simulink library "starslibAirData"  (R2022b)
settings: Solver=ode45  StartTime=0.0  StopTime=10.0  RelTol=1e-3  EnableMultiTasking=on
undefined symbols (not defined in the file): SimIn
libraries: starslibMathOperations x4
settings Model: Creator=eheim  LastModifiedBy=macheson
settings SolverCC: AlgebraicLoopSolver=TrustRegion
settings DataIOCC: LimitDataPoints=on  SaveFormat=Array  SignalLoggingSaveFormat=ModelDataLogs  ReturnWorkspaceOutputs=off
settings OptimizationCC: ExpressionDepthLimit=2147483647  LifeSpan=inf
settings DebuggingCC: UnderspecifiedInitializationDetection=Classic  MergeDetectMultiDrivingBlocksExec=none  SolverPrmCheckMsg=warning  FcnCallInpInsideContextMsg=warning  UnconnectedInputMsg=warning  UnconnectedOutputMsg=warning  UnconnectedLineMsg=warning  StateNameClashWarn=warning  SFUnexpectedBacktrackingDiag=warning  SFNoUnconditionalDefaultTransitionDiag=warning  SFExecutionAtInitializationDiag=none  SFMachineParentedDataDiag=warning  ArithmeticOperatorsInVariantConditions=warning
settings HardwareCC: ProdBitPerPointer=32  ProdBitPerSizeT=32  ProdBitPerPtrDiffT=32  ProdLargestAtomicFloat=None  ProdIntDivRoundTo=Undefined  ProdEndianess=Unspecified  ProdWordSize=32  ProdHWDeviceType=32-bit Generic
settings ModelReferenceCC: PropagateSignalLabelsOutOfModel=off
settings SFSimCC: SimUseLocalCustomCode=off  CustomCodeUndefinedFunction=UseInterfaceOnly
settings RTWCC: RTWUseLocalCustomCode=off
settings CodeAppCC: StateflowObjectComments=on
settings GRTTargetCC: TargetLangStandard=C89/C90 (ANSI)  CombineOutputUpdateFcns=off  GRTInterface=on
settings ConfigComp: CovMetricSettings=dw  CovSaveCumulativeToWorkspaceVar=on  CovSaveSingleToWorkspaceVar=on  CovExternalEMLEnable=off  CovSFcnEnable=off

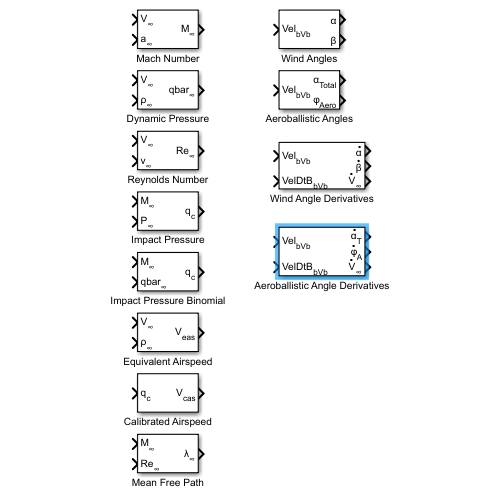
[thumbnail: Simulink's stored preview of the top-level diagram]
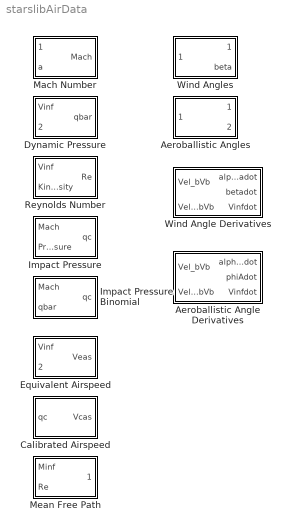
== system starslibAirData ==
  Aeroballistic Angle Derivatives : Subsystem  mask(Aeroballistic Angle Derivatives){}
      mask help: Rate of change of total angle of attack, clocking angle and airspeed with time.
      mask Display:
      | port_label('input' ,1,'Vel_{bVb}','texmode','on')
      | port_label('input' ,2,'VelDtB_{bVb}','texmode','on')
      | port_label('output',1,'\alpha_{T}','texmode','on')
      | text(0.9,1.12,'\fontsize{20}.','texmode', 'on','HorizontalAlignment','Center','VerticalAlignment','Middle')
      | port_label('output',2,'\phi_{A}','texmode','on')
      | text(0.89,0.78,'\fontsize{20}.','texmode', 'on','HorizontalAlignment','Center','VerticalAlignment','Middle')
      | port_label('output',3,'V_{\infty}','texmode','on')
      | text(0.86,0.5,'\fontsize{20}.','texmode', 'on','HorizontalAlignment','Center','VerticalAlignment','Middle')
  Aeroballistic Angles : Subsystem  mask(Aeroballistic Angles){}
      mask help: Total incidence angle (alpha-total) and clocking angle (phi-aero).
      mask Display:
      | port_label('input' ,1,'Vel_{bVb}','texmode','on')
      | port_label('output',1,'\alpha_{Total}','texmode','on')
      | port_label('output',2,'\phi_{Aero}','texmode','on')
  Calibrated Airspeed : Subsystem  mask(Calibrated Airspeed){rhoref=SimIn.Environment.Atmos.rho0, Pref=SimIn.Environment.Atmos.Ps0, gamma=SimIn.Environment.Atmos.gamma}
      mask prompts: rhoref "Standard day sea level density"; Pref "Standard day sea level pressure"; gamma "Ratio of specific heats"
      mask help:
      | Airspeed provided by an ideal airspeed indicator.
      |
      | Units of standard day sea level density and pressure must be consistent with units of impact pressure. The actual standard day sea level density should be derived using standard day pressure and temperature. Typical values are:
      |
      | Pressure 101325 N/m^2 or 29.92 inHg
      | Density 1.2250 kg/m^3 (approximate)
      | Ratio of specific heats 1.4
      mask Display:
      | port_label('input' ,1,'q_c','texmode','on')
      | port_label('output',1,'V_{cas}','texmode','on')
  Dynamic Pressure : Subsystem  mask(Dynamic Pressure){}
      mask help: Local dynamic pressure.
      mask Display:
      | port_label('input' ,1,'V_\infty','texmode','on')
      | port_label('input' ,2,'\rho_\infty','texmode','on')
      | port_label('output',1,'qbar_\infty','texmode','on')
  Equivalent Airspeed : Subsystem  mask(Equivalent Airspeed){rhoref=SimIn.Environment.Atmos.rho0}
      mask prompts: rhoref "Constant sea level density"
      mask help:
      | True airspeed adjusted for standard day density.
      |
      | Units of standard day sea level density and pressure must be consistent with units of impact pressure. The actual standard day sea level density should be derived using standard day pressure and temperature. Typical values are:
      |
      | Density 1.2250 kg/m^3 (approximate)
      mask Display:
      | port_label('input' ,1,'V_\infty','texmode','on')
      | port_label('input' ,2,'\rho_\infty','texmode','on')
      | port_label('output',1,'V_{eas}','texmode','on')
  Impact Pressure : Subsystem  mask(Impact Pressure){gamma=1.4}
      mask prompts: gamma "Ratio of specific heats"
      mask help: Compressible differential pressure.
      mask Display:
      | port_label('input' ,1,'M_\infty','texmode','on')
      | port_label('input' ,2,'P_\infty','texmode','on')
      | port_label('output',1,'q_{c}','texmode','on')
  Impact Pressure Binomial : Subsystem  mask(Impact Pressure Binomial){}
      mask help: Subsonic approximation of impact pressure using binomial expansion.
      mask Display:
      | port_label('input' ,1,'M_\infty','texmode','on')
      | port_label('input' ,2,'qbar_\infty','texmode','on')
      | port_label('output',1,'q_{c}','texmode','on')
  Mach Number : Subsystem  mask(Mach Number){}
      mask help: Ratio of air relative velocity to local speed of sound.
      mask Display:
      | port_label('input' ,1,'V_\infty','texmode','on')
      | port_label('input' ,2,'a_\infty','texmode','on')
      | port_label('output',1,'M_\infty','texmode','on')
  Mean Free Path : Subsystem  mask(Mean Free Path){gamma=1.4}
      mask prompts: gamma "Ratio of specific heats"
      mask help: Average distance between particles.
      mask Display:
      | port_label('input' ,1,'M_\infty','texmode','on')
      | port_label('input' ,2,'Re_\infty','texmode','on')
      | port_label('output',1,'\lambda_\infty','texmode','on')
  Reynolds Number : Subsystem  mask(Reynolds Number){lref=1}
      mask prompts: lref "Reference Length"
      mask help: Local Reynolds Number.
      mask Display:
      | port_label('input' ,1,'V_\infty','texmode','on')
      | port_label('input' ,2,'\nu_\infty','texmode','on')
      | port_label('output',1,'Re_\infty','texmode','on')
  Wind Angle Derivatives : Subsystem  mask(Wind Angle Derivatives){}
      mask help: Rate of change of angle of attack, side slip and airspeed with time.
      mask Display:
      | port_label('input' ,1,'Vel_{bVb}','texmode','on')
      | port_label('input' ,2,'VelDtB_{bVb}','texmode','on')
      | port_label('output',1,'\alpha','texmode','on')
      | text(0.96,1.07,'\fontsize{20}.','texmode', 'on','HorizontalAlignment','Center','VerticalAlignment','Middle')
      | port_label('output',2,'\beta','texmode','on')
      | text(0.95,0.78,'\fontsize{20}.','texmode', 'on','HorizontalAlignment','Center','VerticalAlignment','Middle')
      | port_label('output',3,'V_{\infty}','texmode','on')
      | text(0.86,0.5,'\fontsize{20}.','texmode', 'on','HorizontalAlignment','Center','VerticalAlignment','Middle')
  Wind Angles : Subsystem  mask(Wind Angles){}
      mask help: Angle of attack and sideslip.
      mask Display:
      | port_label('input' ,1,'Vel_{bVb}','texmode','on')
      | port_label('output',1,'\alpha','texmode','on')
      | port_label('output',2,'\beta','texmode','on')

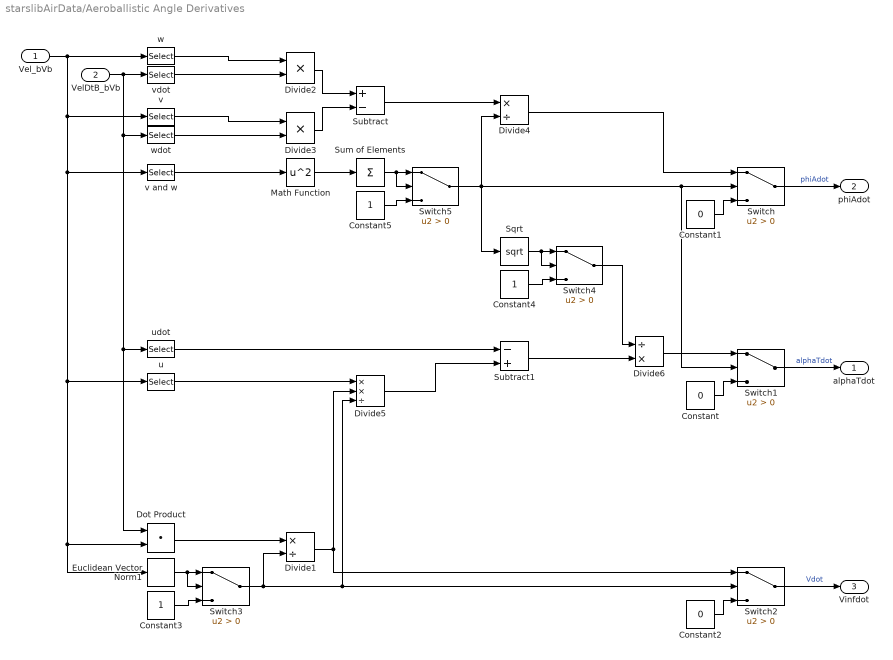
== system starslibAirData/Aeroballistic Angle Derivatives ==
  Vel_bVb : Inport  PortDimensions=[3,1]
  VelDtB_bVb : Inport  Port=2  PortDimensions=[3,1]
  Constant : Constant  Value=0
  Constant1 : Constant  Value=0
  Constant2 : Constant  Value=0
  Constant3 : Constant
  Constant4 : Constant
  Constant5 : Constant
  Divide1 : Product  Inputs=*/
  Divide2 : Product
  Divide3 : Product
  Divide4 : Product  Inputs=*/
  Divide5 : Product  Inputs=**/
  Divide6 : Product  Inputs=/*
  Dot Product : DotProduct  OutDataTypeStr=Inherit: Inherit via internal rule
  Euclidean Vector Norm1 : starslibMathOperations/Euclidean Vector Norm  dim=1
  Math Function : Math  Operator=square  SignedPower=on
  Sqrt : Sqrt
  Subtract : Sum  Inputs=+-
  Subtract1 : Sum  Inputs=-+
  Sum of Elements : Sum  Inputs=+  CollapseMode=Specified dimension
  Switch{,1..5} (6 alike) : Switch  Criteria=u2 > Threshold  SaturateOnIntegerOverflow=off  InputSameDT=off
  u : Selector  NumberOfDimensions=2  InputPortWidth=3  IndexOptions=Index vector (dialog),Select all  Indices=1,1  OutputSizes=1,1
  udot : Selector  NumberOfDimensions=2  InputPortWidth=3  IndexOptions=Index vector (dialog),Select all  Indices=1,1  OutputSizes=1,1
  v : Selector  NumberOfDimensions=2  InputPortWidth=3  IndexOptions=Index vector (dialog),Select all  Indices=2,1  OutputSizes=1,1
  v and w : Selector  NumberOfDimensions=2  InputPortWidth=3  IndexOptions=Index vector (dialog),Select all  Indices=[2 3],1  OutputSizes=1,1
  vdot : Selector  NumberOfDimensions=2  InputPortWidth=3  IndexOptions=Index vector (dialog),Select all  Indices=2,1  OutputSizes=1,1
  w : Selector  NumberOfDimensions=2  InputPortWidth=3  IndexOptions=Index vector (dialog),Select all  Indices=3,1  OutputSizes=1,1
  wdot : Selector  NumberOfDimensions=2  InputPortWidth=3  IndexOptions=Index vector (dialog),Select all  Indices=3,1  OutputSizes=1,1
  alphaTdot : Outport
  phiAdot : Outport  Port=2
  Vinfdot : Outport  Port=3
  wires:
  vdot/1 -> Divide2/2
  w/1 -> Divide2/1
  Vel_bVb/1 -> Euclidean Vector Norm1/1, Dot Product/2, u/1, v and w/1, v/1, w/1
  VelDtB_bVb/1 -> udot/1, Dot Product/1, wdot/1, vdot/1
  Switch2/1 -> Vinfdot/1  "Vdot"
  Constant2/1 -> Switch2/3
  Switch1/1 -> alphaTdot/1  "alphaTdot"
  Constant1/1 -> Switch/3
  Divide6/1 -> Switch1/1
  Subtract1/1 -> Divide6/2
  u/1 -> Divide5/1
  Divide5/1 -> Subtract1/2
  udot/1 -> Subtract1/1
  Divide4/1 -> Switch/1
  Switch5/1 -> Sqrt/1, Divide4/2, Switch1/2, Switch/2
  v and w/1 -> Math Function/1
  Math Function/1 -> Sum of Elements/1
  Subtract/1 -> Divide4/1
  Divide3/1 -> Subtract/2
  Divide2/1 -> Subtract/1
  wdot/1 -> Divide3/2
  v/1 -> Divide3/1
  Divide1/1 -> Switch2/1, Divide5/2
  Switch3/1 -> Divide5/3, Switch2/2, Divide1/2
  Dot Product/1 -> Divide1/1
  Constant/1 -> Switch1/3
  Switch/1 -> phiAdot/1  "phiAdot"
  Constant5/1 -> Switch5/3
  Sum of Elements/1 -> Switch5/2, Switch5/1
  Constant3/1 -> Switch3/3
  Euclidean Vector Norm1/1 -> Switch3/2, Switch3/1
  Constant4/1 -> Switch4/3
  Sqrt/1 -> Switch4/2, Switch4/1
  Switch4/1 -> Divide6/1

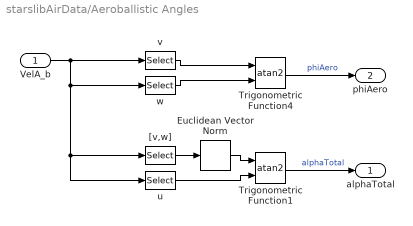
== system starslibAirData/Aeroballistic Angles ==
  VelA_b : Inport
  Euclidean Vector Norm : starslibMathOperations/Euclidean Vector Norm  dim=1
  Trigonometric Function1 : Trigonometry  Operator=atan2  OutputSignalType=real
  Trigonometric Function4 : Trigonometry  Operator=atan2  OutputSignalType=real
  "[v,w]" : Selector  NumberOfDimensions=2  InputPortWidth=3  IndexOptions=Index vector (dialog),Select all  Indices=[2 3],1  OutputSizes=1,1
  u : Selector  NumberOfDimensions=2  InputPortWidth=3  IndexOptions=Index vector (dialog),Select all  Indices=1,1  OutputSizes=1,1
  v : Selector  NumberOfDimensions=2  InputPortWidth=3  IndexOptions=Index vector (dialog),Select all  Indices=2,1  OutputSizes=1,1
  w : Selector  NumberOfDimensions=2  InputPortWidth=3  IndexOptions=Index vector (dialog),Select all  Indices=3,1  OutputSizes=1,1
  alphaTotal : Outport
  phiAero : Outport  Port=2
  wires:
  v/1 -> Trigonometric Function4/1
  w/1 -> Trigonometric Function4/2
  Trigonometric Function4/1 -> phiAero/1  "phiAero"
  Trigonometric Function1/1 -> alphaTotal/1  "alphaTotal"
  Euclidean Vector Norm/1 -> Trigonometric Function1/1
  "[v,w]"/1 -> Euclidean Vector Norm/1
  u/1 -> Trigonometric Function1/2
  VelA_b/1 -> v/1, w/1, "[v,w]"/1, u/1

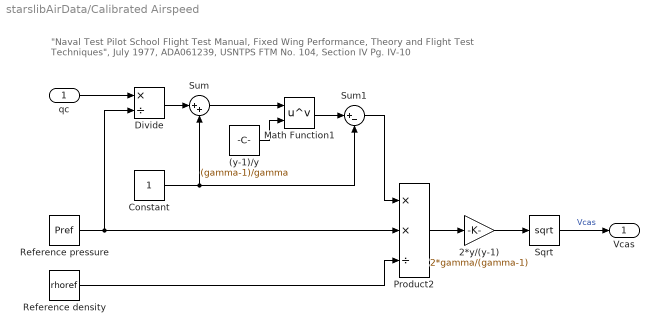
== system starslibAirData/Calibrated Airspeed ==
  note: "Naval Test Pilot School Flight Test Manual, Fixed Wing Performance, Theory and Flight Test Techniques", July 1977, ADA061239, USNTPS FTM No. 104, Section IV Pg. IV-10
  qc : Inport
  (y-1)/y : Constant  Value=(gamma-1)/gamma
  2*y/(y-1) : Gain  Gain=2*gamma/(gamma-1)
  Constant : Constant
  Divide : Product  Inputs=*/
  Math Function1 : Math  Operator=pow  SignedPower=on
  Product2 : Product  Inputs=**/  RndMeth=Zero
  Reference density : Constant  Value=rhoref
  Reference pressure : Constant  Value=Pref
  Sqrt : Sqrt
  Sum : Sum  Inputs=|++
  Sum1 : Sum  Inputs=|+-
  Vcas : Outport
  wires:
  Sqrt/1 -> Vcas/1  "Vcas"
  Reference pressure/1 -> Divide/2, Product2/2
  qc/1 -> Divide/1
  Divide/1 -> Sum/1
  Constant/1 -> Sum/2, Sum1/2
  Sum/1 -> Math Function1/1
  (y-1)/y/1 -> Math Function1/2
  Math Function1/1 -> Sum1/1
  2*y/(y-1)/1 -> Sqrt/1
  Sum1/1 -> Product2/1
  Reference density/1 -> Product2/3
  Product2/1 -> 2*y/(y-1)/1

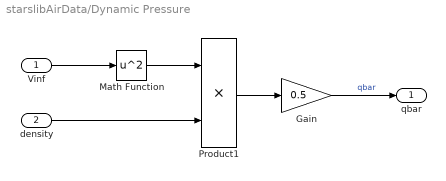
== system starslibAirData/Dynamic Pressure ==
  Vinf : Inport
  density : Inport  Port=2
  Gain : Gain  Gain=0.5  SaturateOnIntegerOverflow=on  OutDataTypeStr=Inherit: Same as input  ParamDataTypeStr=Inherit: Same as input
  Math Function : Math  Operator=square  SignedPower=on
  Product1 : Product  InputSameDT=on  SaturateOnIntegerOverflow=on  OutDataTypeStr=Inherit: Same as first input
  qbar : Outport
  wires:
  Vinf/1 -> Math Function/1
  Product1/1 -> Gain/1
  Gain/1 -> qbar/1  "qbar"
  Math Function/1 -> Product1/1
  density/1 -> Product1/2

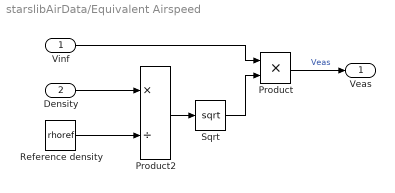
== system starslibAirData/Equivalent Airspeed ==
  Vinf : Inport
  Density : Inport  Port=2
  Product : Product  RndMeth=Zero
  Product2 : Product  Inputs=*/  RndMeth=Zero
  Reference density : Constant  Value=rhoref
  Sqrt : Sqrt
  Veas : Outport
  wires:
  Sqrt/1 -> Product/2
  Product2/1 -> Sqrt/1
  Product/1 -> Veas/1  "Veas"
  Vinf/1 -> Product/1
  Reference density/1 -> Product2/2
  Density/1 -> Product2/1

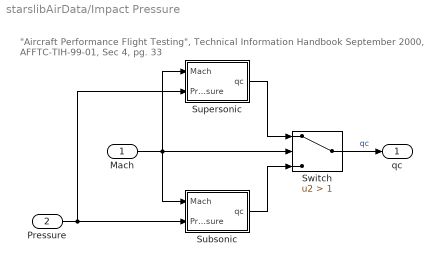
== system starslibAirData/Impact Pressure ==
  note: "Aircraft Performance Flight Testing", Technical Information Handbook September 2000, AFFTC-TIH-99-01, Sec 4, pg. 33
  Mach : Inport
  Pressure : Inport  Port=2
  Subsonic : Subsystem
  Supersonic : Subsystem
  Switch : Switch  Criteria=u2 > Threshold  Threshold=1  SaturateOnIntegerOverflow=off  InputSameDT=off
  qc : Outport
  wires:
  Mach/1 -> Subsonic/1(Mach), Switch/2, Supersonic/1(Mach)
  Pressure/1 -> Subsonic/2(Pressure), Supersonic/2(Pressure)
  Supersonic/1(qc) -> Switch/1
  Subsonic/1(qc) -> Switch/3
  Switch/1 -> qc/1  "qc"

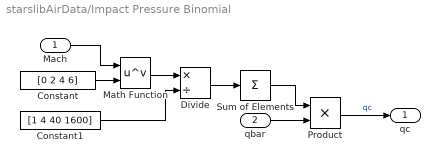
== system starslibAirData/Impact Pressure Binomial ==
  Mach : Inport
  qbar : Inport  Port=2
  Constant : Constant  Value=[0 2 4 6]
  Constant1 : Constant  Value=[1 4 40 1600]
  Divide : Product  Inputs=*/
  Math Function : Math  Operator=pow  SignedPower=on
  Product : Product  RndMeth=Zero
  Sum of Elements : Sum  Inputs=+
  qc : Outport
  wires:
  Math Function/1 -> Divide/1
  Divide/1 -> Sum of Elements/1
  Constant/1 -> Math Function/2
  Constant1/1 -> Divide/2
  Mach/1 -> Math Function/1
  Sum of Elements/1 -> Product/1
  qbar/1 -> Product/2
  Product/1 -> qc/1  "qc"

== system starslibAirData/Mach Number ==
  Vtotal : Inport
  a : Inport  Port=2
  Product2 : Product  Inputs=*/  SaturateOnIntegerOverflow=on  OutDataTypeStr=Inherit: Same as first input
  Mach : Outport
  wires:
  a/1 -> Product2/2
  Product2/1 -> Mach/1  "Mach"
  Vtotal/1 -> Product2/1

== system starslibAirData/Mean Free Path ==
  Minf : Inport
  Re : Inport  Port=2
  Product1 : Product  Inputs=**/  InputSameDT=on  SaturateOnIntegerOverflow=on  OutDataTypeStr=Inherit: Same as first input
  sqrt(gamma*pi/2) : Constant  Value=sqrt(gamma*pi/2)
  mean free path : Outport
  wires:
  Re/1 -> Product1/3
  sqrt(gamma*pi/2)/1 -> Product1/2
  Minf/1 -> Product1/1
  Product1/1 -> mean free path/1  "mfp"

== system starslibAirData/Reynolds Number ==
  Vinf : Inport
  Kinematic viscosity : Inport  Port=2
  Product1 : Product  Inputs=**/  InputSameDT=on  SaturateOnIntegerOverflow=on  OutDataTypeStr=Inherit: Same as first input
  Reference length : Constant  Value=lref
  Re : Outport
  wires:
  Product1/1 -> Re/1  "Re"
  Vinf/1 -> Product1/1
  Reference length/1 -> Product1/2
  Kinematic viscosity/1 -> Product1/3

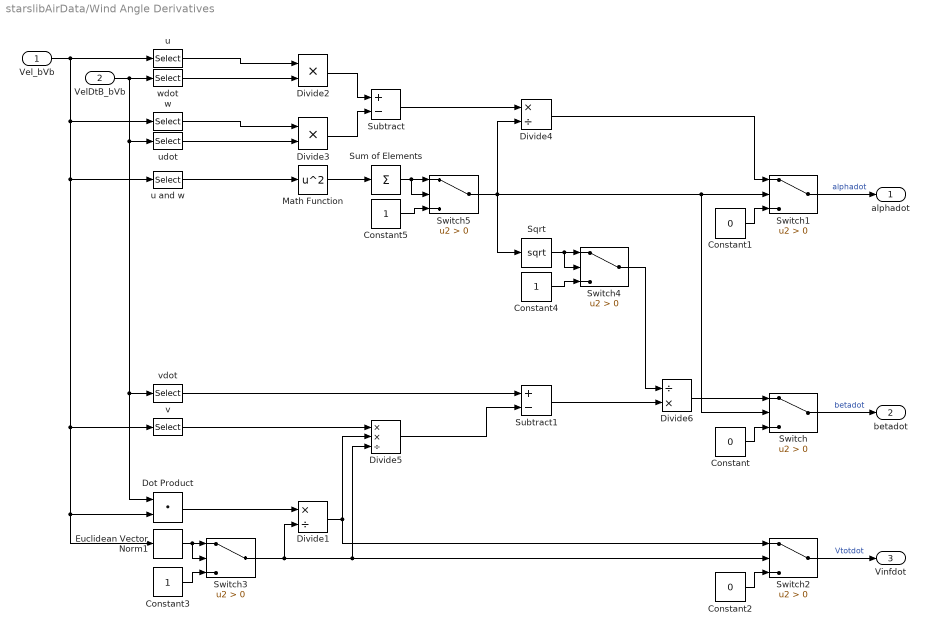
== system starslibAirData/Wind Angle Derivatives ==
  Vel_bVb : Inport  PortDimensions=[3,1]
  VelDtB_bVb : Inport  Port=2  PortDimensions=[3,1]
  Constant : Constant  Value=0
  Constant1 : Constant  Value=0
  Constant2 : Constant  Value=0
  Constant3 : Constant
  Constant4 : Constant
  Constant5 : Constant
  Divide1 : Product  Inputs=*/
  Divide2 : Product
  Divide3 : Product
  Divide4 : Product  Inputs=*/
  Divide5 : Product  Inputs=**/
  Divide6 : Product  Inputs=/*
  Dot Product : DotProduct  OutDataTypeStr=Inherit: Inherit via internal rule
  Euclidean Vector Norm1 : starslibMathOperations/Euclidean Vector Norm  dim=1
  Math Function : Math  Operator=square  SignedPower=on
  Sqrt : Sqrt
  Subtract : Sum  Inputs=+-
  Subtract1 : Sum  Inputs=+-
  Sum of Elements : Sum  Inputs=+  CollapseMode=Specified dimension
  Switch{,1..5} (6 alike) : Switch  Criteria=u2 > Threshold  SaturateOnIntegerOverflow=off  InputSameDT=off
  u : Selector  NumberOfDimensions=2  InputPortWidth=3  IndexOptions=Index vector (dialog),Select all  Indices=1,1  OutputSizes=1,1
  u and w : Selector  NumberOfDimensions=2  InputPortWidth=3  IndexOptions=Index vector (dialog),Select all  Indices=[1 3],1  OutputSizes=1,1
  udot : Selector  NumberOfDimensions=2  InputPortWidth=3  IndexOptions=Index vector (dialog),Select all  Indices=1,1  OutputSizes=1,1
  v : Selector  NumberOfDimensions=2  InputPortWidth=3  IndexOptions=Index vector (dialog),Select all  Indices=2,1  OutputSizes=1,1
  vdot : Selector  NumberOfDimensions=2  InputPortWidth=3  IndexOptions=Index vector (dialog),Select all  Indices=2,1  OutputSizes=1,1
  w : Selector  NumberOfDimensions=2  InputPortWidth=3  IndexOptions=Index vector (dialog),Select all  Indices=3,1  OutputSizes=1,1
  wdot : Selector  NumberOfDimensions=2  InputPortWidth=3  IndexOptions=Index vector (dialog),Select all  Indices=3,1  OutputSizes=1,1
  alphadot : Outport
  betadot : Outport  Port=2
  Vinfdot : Outport  Port=3
  wires:
  Switch/1 -> betadot/1  "betadot"
  Constant/1 -> Switch/3
  Dot Product/1 -> Divide1/1
  Switch3/1 -> Divide1/2, Divide5/3, Switch2/2
  Divide1/1 -> Divide5/2, Switch2/1
  w/1 -> Divide3/1
  udot/1 -> Divide3/2
  Divide2/1 -> Subtract/1
  Divide3/1 -> Subtract/2
  Subtract/1 -> Divide4/1
  Math Function/1 -> Sum of Elements/1
  u and w/1 -> Math Function/1
  Switch5/1 -> Switch1/2, Switch/2, Divide4/2, Sqrt/1
  Divide4/1 -> Switch1/1
  vdot/1 -> Subtract1/1
  Divide5/1 -> Subtract1/2
  v/1 -> Divide5/1
  Subtract1/1 -> Divide6/2
  Divide6/1 -> Switch/1
  Constant1/1 -> Switch1/3
  Switch1/1 -> alphadot/1  "alphadot"
  Constant2/1 -> Switch2/3
  Switch2/1 -> Vinfdot/1  "Vtotdot"
  VelDtB_bVb/1 -> wdot/1, udot/1, vdot/1, Dot Product/1
  Vel_bVb/1 -> u/1, w/1, u and w/1, v/1, Euclidean Vector Norm1/1, Dot Product/2
  u/1 -> Divide2/1
  wdot/1 -> Divide2/2
  Constant3/1 -> Switch3/3
  Euclidean Vector Norm1/1 -> Switch3/2, Switch3/1
  Constant4/1 -> Switch4/3
  Sqrt/1 -> Switch4/1, Switch4/2
  Switch4/1 -> Divide6/1
  Constant5/1 -> Switch5/3
  Sum of Elements/1 -> Switch5/2, Switch5/1

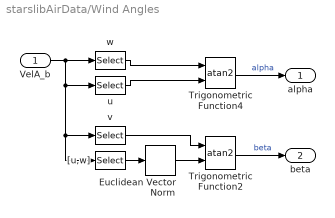
== system starslibAirData/Wind Angles ==
  VelA_b : Inport
  Euclidean Vector Norm : starslibMathOperations/Euclidean Vector Norm  dim=1
  Trigonometric Function2 : Trigonometry  Operator=atan2  OutputSignalType=real
  Trigonometric Function4 : Trigonometry  Operator=atan2  OutputSignalType=real
  "[u,w]" : Selector  NumberOfDimensions=2  InputPortWidth=3  IndexOptions=Index vector (dialog),Select all  Indices=[1 3],1  OutputSizes=1,1
  u : Selector  NumberOfDimensions=2  InputPortWidth=3  IndexOptions=Index vector (dialog),Select all  Indices=1,1  OutputSizes=1,1
  v : Selector  NumberOfDimensions=2  InputPortWidth=3  IndexOptions=Index vector (dialog),Select all  Indices=2,1  OutputSizes=1,1
  w : Selector  NumberOfDimensions=2  InputPortWidth=3  IndexOptions=Index vector (dialog),Select all  Indices=3,1  OutputSizes=1,1
  alpha : Outport
  beta : Outport  Port=2
  wires:
  Trigonometric Function2/1 -> beta/1  "beta"
  Trigonometric Function4/1 -> alpha/1  "alpha"
  u/1 -> Trigonometric Function4/2
  w/1 -> Trigonometric Function4/1
  Euclidean Vector Norm/1 -> Trigonometric Function2/2
  v/1 -> Trigonometric Function2/1
  "[u,w]"/1 -> Euclidean Vector Norm/1
  VelA_b/1 -> w/1, u/1, v/1, "[u,w]"/1

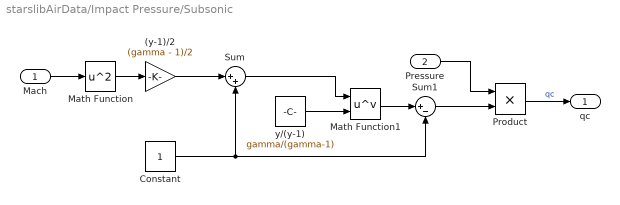
== system starslibAirData/Impact Pressure/Subsonic ==
  Mach : Inport
  Pressure : Inport  Port=2
  (y-1)/2 : Gain  Gain=(gamma - 1)/2
  Constant : Constant
  Math Function : Math  Operator=square  SignedPower=on
  Math Function1 : Math  Operator=pow  SignedPower=on
  Product : Product  RndMeth=Zero
  Sum : Sum  Inputs=|++
  Sum1 : Sum  Inputs=|+-
  y/(y-1) : Constant  Value=gamma/(gamma-1)
  qc : Outport
  wires:
  Mach/1 -> Math Function/1
  Math Function/1 -> (y-1)/2/1
  (y-1)/2/1 -> Sum/1
  Constant/1 -> Sum/2, Sum1/2
  Sum/1 -> Math Function1/1
  y/(y-1)/1 -> Math Function1/2
  Math Function1/1 -> Sum1/1
  Sum1/1 -> Product/2
  Pressure/1 -> Product/1
  Product/1 -> qc/1  "qc"

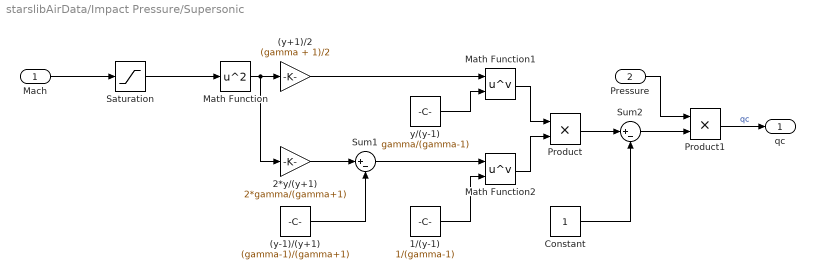
== system starslibAirData/Impact Pressure/Supersonic ==
  Mach : Inport
  Pressure : Inport  Port=2
  (y+1)/2 : Gain  Gain=(gamma + 1)/2
  (y-1)/(y+1) : Constant  Value=(gamma-1)/(gamma+1)
  1/(y-1) : Constant  Value=1/(gamma-1)
  2*y/(y+1) : Gain  Gain=2*gamma/(gamma+1)
  Constant : Constant
  Math Function : Math  Operator=square  SignedPower=on
  Math Function1 : Math  Operator=pow  SignedPower=on
  Math Function2 : Math  Operator=pow  SignedPower=on
  Product : Product  RndMeth=Zero
  Product1 : Product  RndMeth=Zero
  Saturation : Saturate  UpperLimit=Inf  LowerLimit=1  LinearizeAsGain=off
  Sum1 : Sum  Inputs=|+-
  Sum2 : Sum  Inputs=|+-
  y/(y-1) : Constant  Value=gamma/(gamma-1)
  qc : Outport
  wires:
  Product1/1 -> qc/1  "qc"
  y/(y-1)/1 -> Math Function1/2
  (y+1)/2/1 -> Math Function1/1
  Math Function/1 -> (y+1)/2/1, 2*y/(y+1)/1
  Mach/1 -> Saturation/1
  2*y/(y+1)/1 -> Sum1/1
  (y-1)/(y+1)/1 -> Sum1/2
  Sum1/1 -> Math Function2/1
  1/(y-1)/1 -> Math Function2/2
  Math Function1/1 -> Product/1
  Math Function2/1 -> Product/2
  Product/1 -> Sum2/1
  Constant/1 -> Sum2/2
  Sum2/1 -> Product1/2
  Pressure/1 -> Product1/1
  Saturation/1 -> Math Function/1
